simulink model "AMR_Testing_AutoMode_StateFlow"  (R2023b)
settings: Solver=FixedStepAuto  StartTime=0.0  StopTime=150  FixedStep=5e-3  RelTol=1e-3
model workspace (MAT data in the model file):
  RTK_health_condition = 30
  mdlWSDbList = ["C:\Users\matlab.cut\Desktop\AMR\canbus_files\tramontina_database_sick_modbus.dbc" "C:\Users\matlab.cut\Desktop\AMR\canbus_files\tramontina_database_xsens.dbc" "tramontina_database_curtis.dbc"]
  wheel_diameter = 360
  wheel_radius = 180
undefined symbols (not defined in the file or in its folder): Down, Pull
libraries: tramontina_database_xsenslib x4, speedgoatlib_IO60X_IO69X x2, tramontina_database_sick_modbuslib x1, speedgoatlib_IO691 x1, simulink_extras x1
settings Model: Creator=matlab.cut  LastModifiedBy=matlab.cut

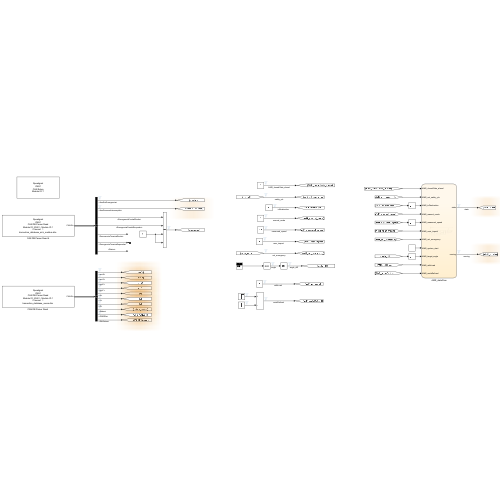
[thumbnail: Simulink's stored preview of the top-level diagram]
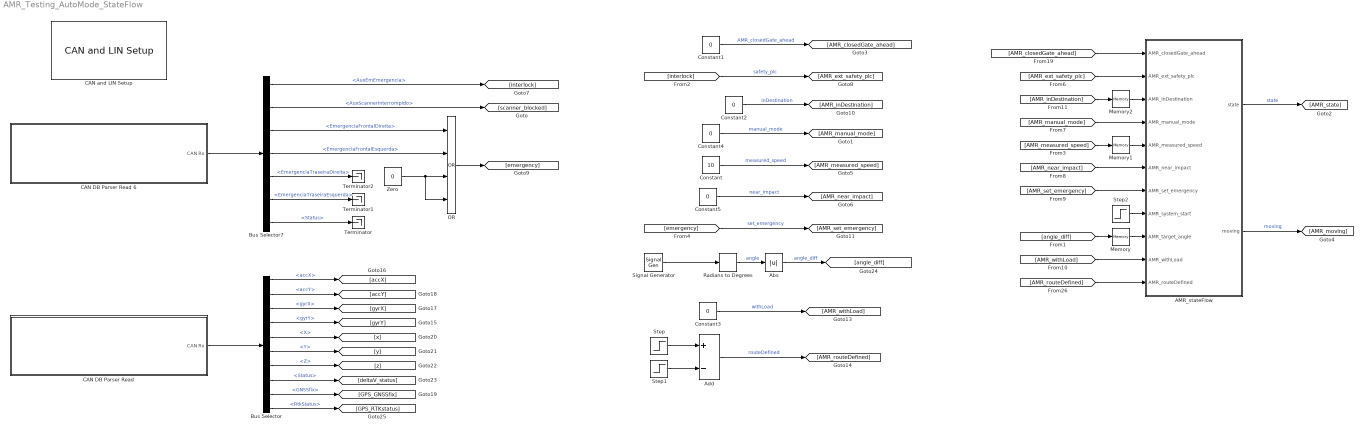
== system AMR_Testing_AutoMode_StateFlow ==
  AMR_stateFlow : Stateflow chart  TreatAsAtomicUnit=on
  Abs : Abs  SaturateOnIntegerOverflow=off
  Add : Sum  Inputs=+-
  Bus Selector : BusSelector  OutputSignals=ID52_Acceleration.accX,ID52_Acceleration.accY,ID50_RateOfTurn.gyrX,ID50_RateOfTurn.gyrY,ID49_DeltaV.X,ID49_DeltaV.Y,ID49_DeltaV.Z,ID49_DeltaV.MessageStatus.Status,ID17_StatusWord.GNSSfix,ID17_StatusWord.RtkStatus
  Bus Selector7 : BusSelector  OutputSignals=ID341_read_from_flexisoft.AuxEmEmergencia,ID341_read_from_flexisoft.AuxScannerInterrompido,ID341_read_from_flexisoft.EmergenciaFrontalDireita,ID341_read_from_flexisoft.EmergenciaFrontalEsquerda,ID341_read_from_flexisoft.EmergenciaTraseiraDireita,ID341_read_from_flexisoft.EmergenciaTraseiraEsquerda,ID341_read_from_flexisoft.MessageStatus.Status
  "CAN DB Parser Read " : Subsystem
      settings: OpenFcn=sg_can.OpenFcnRead;
      mask Help: eval('sg.utils.help.show(''io_main/refentry_ref_can_ofa_parsing_read'');')
      mask Display: disp('Speedgoat\nIO691\nCAN DB Parser Read\nModule ID: IO691 - Module ID 1\nChannel:  1\ntramontina_database_xsens.dbc ');
  CAN DB Parser Read 6 : Subsystem
      settings: OpenFcn=sg_can.OpenFcnRead;
      mask Help: eval('sg.utils.help.show(''io_main/refentry_ref_can_ofa_parsing_read'');')
      mask Display: disp('Speedgoat\nIO691\nCAN DB Parser Read\nModule ID: IO691 - Module ID 1\nChannel:  1\ntramontina_database_sick_modbus.dbc ');
  "CAN and LIN Setup " : speedgoatlib_IO691/CAN and LIN Setup   moduleInitValues="[691    1    1   -1   -1]"  id=1  moduleType=IO691  pciSlot=-1  canChn1=CAN (HS)  canChn2=Disabled  canChn3=Disabled  canChn4=Disabled  linChn1=Disabled  linChn2=Disabled  canInitStructArray=[]  canTermStructArray=[]  gpioChnx=Disabled  canChn1InitValues="[2   2   8   1  16   3  19   2   2   5   2   0]"  arbBdrChn1=500 kBaud  clockDividerChn1=Enable  arbManBdrChn1=[8,1,16,3]  fdBdrChn1=5.0 MBaud  fdManBdrChn1=[2,2,5,2]  termResistor1=off  canChn2InitValues="[1   0   2   8  31   8  19   2   2   5   2   0]"  arbBdrChn2=1.0 MBaud  clockDividerChn2=Enable  arbManBdrChn2=[2,8,31,8]  fdBdrChn2=5.0 MBaud  fdManBdrChn2=[2,2,5,2]  termResistor2=off  canChn3InitValues="[1   0   2   8  31   8  19   2   2   5   2   0]"  arbBdrChn3=1.0 MBaud  clockDividerChn3=Enable  arbManBdrChn3=[2,8,31,8]  fdBdrChn3=5.0 MBaud  fdManBdrChn3=[2,2,5,2]  termResistor3=off  canChn4InitValues="[1   0   2   8  31   8  19   2   2   5   2   0]"  arbBdrChn4=1.0 MBaud  clockDividerChn4=Enable  arbManBdrChn4=[2,8,31,8]  fdBdrChn4=5.0 MBaud  fdManBdrChn4=[2,2,5,2]  termResistor4=off  linChn1InitValues="[0  9600]"  linBtrChn1=9600  linChn2InitValues="[0  9600]"  linBtrChn2=9600  doInitTermStruct="[0  5  0  0  0]"  parDoChannels=[1 2]  parDoVoltage=5  parDoInitValues=0  parDoReset=1  parNumOfDoS=0  parDiChannels=[3 4]  parDiVoltage=5  parDiPull=Pull-Down
      settings: LibrarySourceBlock=speedgoatlib_IO602_IO691/CAN and LIN Setup
  Constant : Constant  Value=10
  Constant{1..5} (5 alike) : Constant  Value=0
  Memory : Memory
  Memory1 : Memory
  Memory2 : Memory
  OR : Logic  Operator=OR  Inputs=4  AllPortsSameDT=off  OutDataTypeStr=boolean
  Radians to Degrees : simulink_extras/Transformations/Radians to Degrees
  Signal Generator : SignalGenerator  Amplitude=0.1  Frequency=0.5
  Step : Step  Time=15  SampleTime=0
  Step1 : Step  Time=20  SampleTime=0
  Step2 : Step  Time=5  SampleTime=0
  Terminator : Terminator
  Terminator1 : Terminator
  Terminator2 : Terminator
  Zero : Constant  Value=0  OutDataTypeStr=Inherit: Inherit via back propagation
  wires:
  Memory/1 -> AMR_stateFlow/9(AMR_target_angle)
  Memory1/1 -> AMR_stateFlow/5(AMR_measured_speed)
  Step2/1 -> AMR_stateFlow/8(AMR_system_start)
  Memory2/1 -> AMR_stateFlow/3(AMR_inDestination)
  [AMR_routeDefined] -> AMR_stateFlow/11(AMR_routeDefined)
  [angle_diff] -> Memory/1
  [AMR_inDestination] -> Memory2/1
  [AMR_manual_mode] -> AMR_stateFlow/4(AMR_manual_mode)
  [AMR_near_impact] -> AMR_stateFlow/6(AMR_near_impact)
  [AMR_closedGate_ahead] -> AMR_stateFlow/1(AMR_closedGate_ahead)
  [AMR_measured_speed] -> Memory1/1
  AMR_stateFlow/2(moving) -> [AMR_moving]  "moving"
  [AMR_withLoad] -> AMR_stateFlow/10(AMR_withLoad)
  AMR_stateFlow/1(state) -> [AMR_state]  "state"
  [AMR_set_emergency] -> AMR_stateFlow/7(AMR_set_emergency)
  [AMR_ext_safety_plc] -> AMR_stateFlow/2(AMR_ext_safety_plc)
  Constant4/1 -> [AMR_manual_mode]  "manual_mode"
  Constant/1 -> [AMR_measured_speed]  "measured_speed"
  Constant5/1 -> [AMR_near_impact]  "near_impact"
  [interlock] -> [AMR_ext_safety_plc]  "safety_plc"
  Constant1/1 -> [AMR_closedGate_ahead]  "AMR_closedGate_ahead"
  Constant2/1 -> [AMR_inDestination]  "inDestination"
  [emergency] -> [AMR_set_emergency]  "set_emergency"
  Constant3/1 -> [AMR_withLoad]  "withLoad"
  Add/1 -> [AMR_routeDefined]  "routeDefined"
  Bus Selector7/5 -> Terminator2/1  "<EmergenciaTraseiraDireita>"
  Zero/1 -> OR/4, OR/3
  Bus Selector7/4 -> OR/2  "<EmergenciaFrontalEsquerda>"
  CAN DB Parser Read 6/1(CAN Rx) -> Bus Selector7/1
  Bus Selector7/7 -> Terminator/1  "<Status>"
  Bus Selector7/2 -> [scanner_blocked]  "<AuxScannerInterrompido>"
  Bus Selector7/6 -> Terminator1/1  "<EmergenciaTraseiraEsquerda>"
  Bus Selector7/3 -> OR/1  "<EmergenciaFrontalDireita>"
  Bus Selector7/1 -> [interlock]  "<AuxEmEmergencia>"
  OR/1 -> [emergency]
  Step1/1 -> Add/2
  Step/1 -> Add/1
  Bus Selector/10 -> [GPS_RTKstatus]  "<RtkStatus>"
  "CAN DB Parser Read "/1(CAN Rx) -> Bus Selector/1
  Bus Selector/3 -> [gyrX]  "<gyrX>"
  Bus Selector/2 -> [accY]  "<accY>"
  Bus Selector/4 -> [gyrY]  "<gyrY>"
  Bus Selector/1 -> [accX]  "<accX>"
  Bus Selector/9 -> [GPS_GNSSfix]  "<GNSSfix>"
  Bus Selector/5 -> [x]  "<X>"
  Bus Selector/6 -> [y]  "<Y>"
  Bus Selector/7 -> [z]  "<Z>"
  Bus Selector/8 -> [deltaV_status]  "<Status>"
  Abs/1 -> [angle_diff]  "angle_diff"
  Signal Generator/1 -> Radians to Degrees/1
  Radians to Degrees/1 -> Abs/1  "angle"

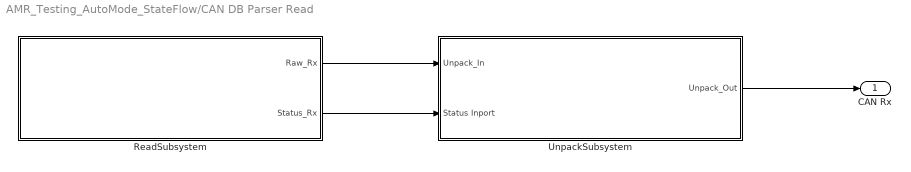
== system AMR_Testing_AutoMode_StateFlow/CAN DB Parser Read  ==
  ReadSubsystem : Subsystem
  UnpackSubsystem : Subsystem
  CAN Rx : Outport
  wires:
  ReadSubsystem/1(Raw_Rx) -> UnpackSubsystem/1(Unpack_In)
  ReadSubsystem/2(Status_Rx) -> UnpackSubsystem/2(Status Inport)
  UnpackSubsystem/1(Unpack_Out) -> CAN Rx/1

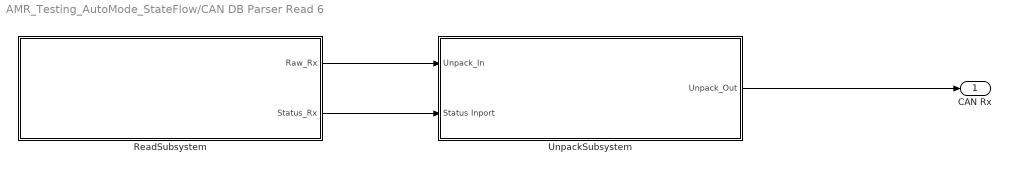
== system AMR_Testing_AutoMode_StateFlow/CAN DB Parser Read 6 ==
  ReadSubsystem : Subsystem
  UnpackSubsystem : Subsystem
  CAN Rx : Outport
  wires:
  ReadSubsystem/1(Raw_Rx) -> UnpackSubsystem/1(Unpack_In)
  ReadSubsystem/2(Status_Rx) -> UnpackSubsystem/2(Status Inport)
  UnpackSubsystem/1(Unpack_Out) -> CAN Rx/1

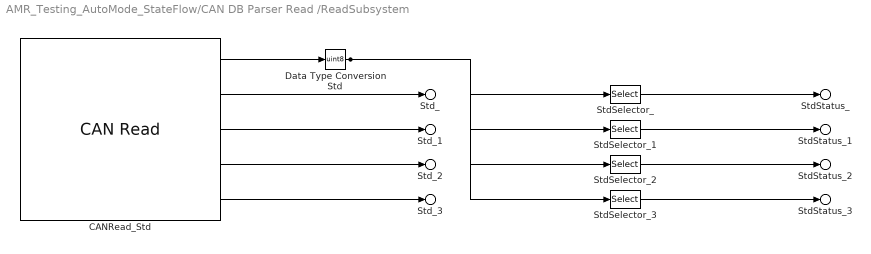
== system AMR_Testing_AutoMode_StateFlow/CAN DB Parser Read /ReadSubsystem ==
  CANRead_Std : speedgoatlib_IO60X_IO69X/CAN/CAN Read   moduleType=IO691  id=1  channel=1  canType=CAN (HS)  messageType=CAN (HS)  useBusOut=on  HasMulRead=Specify by IDs  MsgIDlist="[17  49  50  52]"  isEFF=off  LabelInHex=off  enableInput=off  initValues=[691 1 0.01 0 1 1 0 1 2 0 4 17 49 50 52]  ts=10e-3
  Data Type ConversionStd : DataTypeConversion  OutDataTypeStr=uint8  SaturateOnIntegerOverflow=off  RndMeth=Floor
  StdSelector_ : Selector  IndexOptions=Index vector (dialog)  Indices=1  OutputSizes=1
  StdSelector_1 : Selector  IndexOptions=Index vector (dialog)  Indices=2  OutputSizes=1
  StdSelector_2 : Selector  IndexOptions=Index vector (dialog)  Indices=3  OutputSizes=1
  StdSelector_3 : Selector  IndexOptions=Index vector (dialog)  Indices=4  OutputSizes=1
  Std_ : Outport  PortName=Raw_Rx  Element=Std.ID17
  Std_1 : Outport  PortName=Raw_Rx  Element=Std.ID49
  Std_2 : Outport  PortName=Raw_Rx  Element=Std.ID50
  Std_3 : Outport  PortName=Raw_Rx  Element=Std.ID52
  StdStatus_ : Outport  Port=2  PortName=Status_Rx  Element=Std.ID17
  StdStatus_1 : Outport  Port=2  PortName=Status_Rx  Element=Std.ID49
  StdStatus_2 : Outport  Port=2  PortName=Status_Rx  Element=Std.ID50
  StdStatus_3 : Outport  Port=2  PortName=Status_Rx  Element=Std.ID52
  wires:
  CANRead_Std/1 -> Data Type ConversionStd/1
  CANRead_Std/2 -> Std_/1
  CANRead_Std/3 -> Std_1/1
  CANRead_Std/4 -> Std_2/1
  CANRead_Std/5 -> Std_3/1
  Data Type ConversionStd/1 -> StdSelector_/1, StdSelector_1/1, StdSelector_2/1, StdSelector_3/1
  StdSelector_/1 -> StdStatus_/1
  StdSelector_1/1 -> StdStatus_1/1
  StdSelector_2/1 -> StdStatus_2/1
  StdSelector_3/1 -> StdStatus_3/1

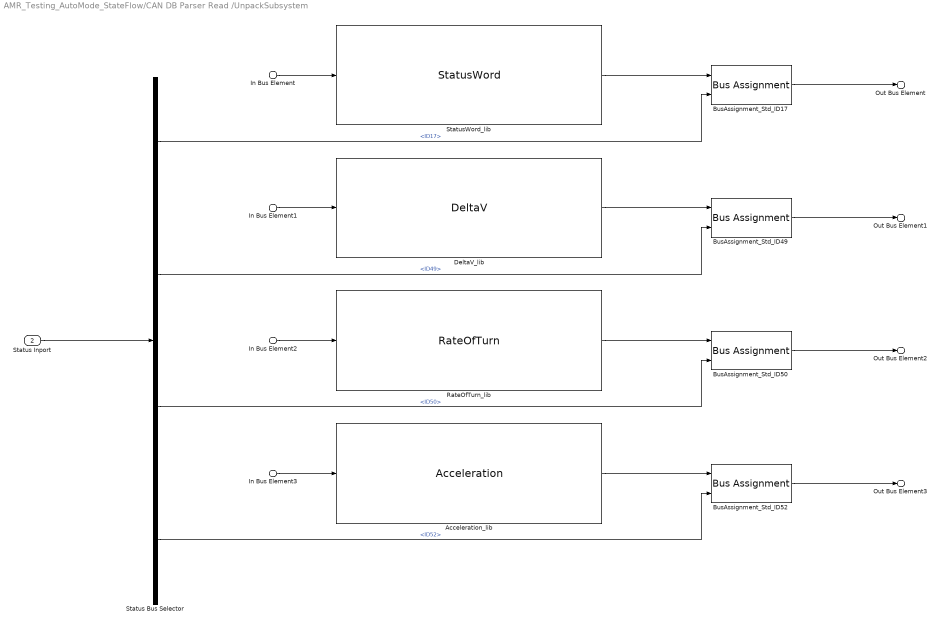
== system AMR_Testing_AutoMode_StateFlow/CAN DB Parser Read /UnpackSubsystem ==
  In Bus Element : Inport  PortName=Unpack_In  Element=Std.ID17
  In Bus Element1 : Inport  PortName=Unpack_In  Element=Std.ID49
  In Bus Element2 : Inport  PortName=Unpack_In  Element=Std.ID50
  In Bus Element3 : Inport  PortName=Unpack_In  Element=Std.ID52
  Status Inport : Inport  Port=2
  Acceleration_lib : tramontina_database_xsenslib/CAN unpack/Acceleration  SystemSampleTime=-1  VariantActivationTime=update diagram  AllowFlexibleInterface=on  Latency=0  AutoFrameSizeCalculation=off
  BusAssignment_Std_ID{17,49..50,52} (4 alike) : BusAssignment  AssignedSignals=MessageStatus.Status
  DeltaV_lib : tramontina_database_xsenslib/CAN unpack/DeltaV  SystemSampleTime=-1  VariantActivationTime=update diagram  AllowFlexibleInterface=on  Latency=0  AutoFrameSizeCalculation=off
  RateOfTurn_lib : tramontina_database_xsenslib/CAN unpack/RateOfTurn  SystemSampleTime=-1  VariantActivationTime=update diagram  AllowFlexibleInterface=on  Latency=0  AutoFrameSizeCalculation=off
  Status Bus Selector : BusSelector  OutputSignals=Std.ID17,Std.ID49,Std.ID50,Std.ID52
  StatusWord_lib : tramontina_database_xsenslib/CAN unpack/StatusWord  SystemSampleTime=-1  VariantActivationTime=update diagram  AllowFlexibleInterface=on  Latency=0  AutoFrameSizeCalculation=off
  Out Bus Element : Outport  PortName=Unpack_Out  Element=ID17_StatusWord
  Out Bus Element1 : Outport  PortName=Unpack_Out  Element=ID49_DeltaV
  Out Bus Element2 : Outport  PortName=Unpack_Out  Element=ID50_RateOfTurn
  Out Bus Element3 : Outport  PortName=Unpack_Out  Element=ID52_Acceleration
  wires:
  In Bus Element/1 -> StatusWord_lib/1
  StatusWord_lib/1 -> BusAssignment_Std_ID17/1
  BusAssignment_Std_ID17/1 -> Out Bus Element/1
  In Bus Element1/1 -> DeltaV_lib/1
  DeltaV_lib/1 -> BusAssignment_Std_ID49/1
  BusAssignment_Std_ID49/1 -> Out Bus Element1/1
  In Bus Element2/1 -> RateOfTurn_lib/1
  RateOfTurn_lib/1 -> BusAssignment_Std_ID50/1
  BusAssignment_Std_ID50/1 -> Out Bus Element2/1
  In Bus Element3/1 -> Acceleration_lib/1
  Acceleration_lib/1 -> BusAssignment_Std_ID52/1
  BusAssignment_Std_ID52/1 -> Out Bus Element3/1
  Status Inport/1 -> Status Bus Selector/1
  Status Bus Selector/1 -> BusAssignment_Std_ID17/2  "<ID17>"
  Status Bus Selector/2 -> BusAssignment_Std_ID49/2  "<ID49>"
  Status Bus Selector/3 -> BusAssignment_Std_ID50/2  "<ID50>"
  Status Bus Selector/4 -> BusAssignment_Std_ID52/2  "<ID52>"

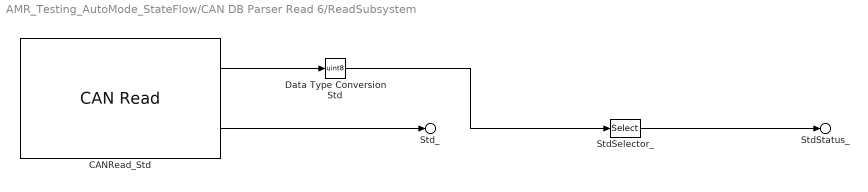
== system AMR_Testing_AutoMode_StateFlow/CAN DB Parser Read 6/ReadSubsystem ==
  CANRead_Std : speedgoatlib_IO60X_IO69X/CAN/CAN Read   moduleType=IO691  id=1  channel=1  canType=CAN (HS)  messageType=CAN (HS)  useBusOut=on  HasMulRead=Specify by IDs  MsgIDlist=[341]  isEFF=off  LabelInHex=off  enableInput=off  initValues=[691 1 0.1 0 1 1 0 1 2 0 1 341]  ts=100e-3
  Data Type ConversionStd : DataTypeConversion  OutDataTypeStr=uint8  SaturateOnIntegerOverflow=off  RndMeth=Floor
  StdSelector_ : Selector  IndexOptions=Index vector (dialog)  Indices=1  OutputSizes=1
  Std_ : Outport  PortName=Raw_Rx  Element=Std.ID341
  StdStatus_ : Outport  Port=2  PortName=Status_Rx  Element=Std.ID341
  wires:
  CANRead_Std/1 -> Data Type ConversionStd/1
  CANRead_Std/2 -> Std_/1
  Data Type ConversionStd/1 -> StdSelector_/1
  StdSelector_/1 -> StdStatus_/1

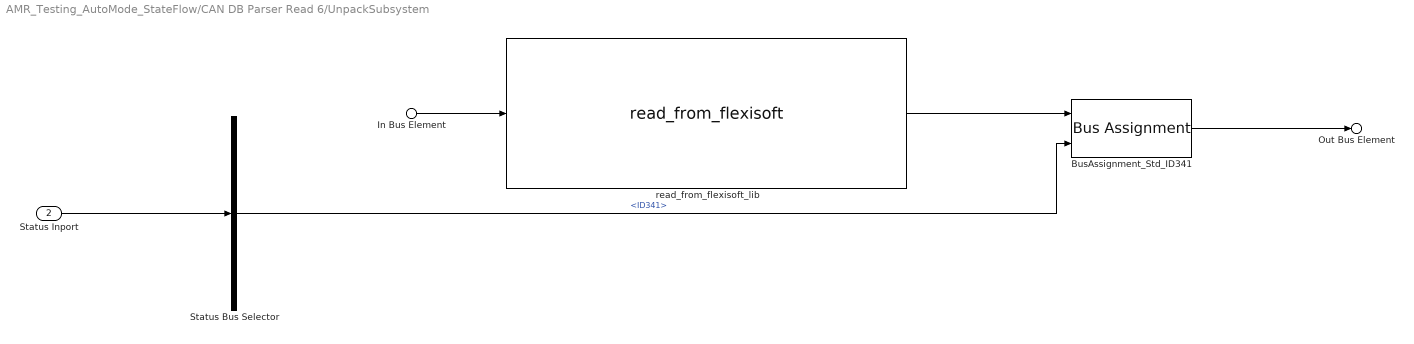
== system AMR_Testing_AutoMode_StateFlow/CAN DB Parser Read 6/UnpackSubsystem ==
  In Bus Element : Inport  PortName=Unpack_In  Element=Std.ID341
  Status Inport : Inport  Port=2
  BusAssignment_Std_ID341 : BusAssignment  AssignedSignals=MessageStatus.Status
  Status Bus Selector : BusSelector  OutputSignals=Std.ID341
  read_from_flexisoft_lib : tramontina_database_sick_modbuslib/CAN unpack/read_from_flexisoft  SystemSampleTime=-1  VariantActivationTime=update diagram  AllowFlexibleInterface=on  Latency=0  AutoFrameSizeCalculation=off
  Out Bus Element : Outport  PortName=Unpack_Out  Element=ID341_read_from_flexisoft
  wires:
  In Bus Element/1 -> read_from_flexisoft_lib/1
  read_from_flexisoft_lib/1 -> BusAssignment_Std_ID341/1
  BusAssignment_Std_ID341/1 -> Out Bus Element/1
  Status Inport/1 -> Status Bus Selector/1
  Status Bus Selector/1 -> BusAssignment_Std_ID341/2  "<ID341>"

== stateflow chart AMR_Testing_AutoMode_StateFlow/AMR_stateFlow ==
  note: Constantes:
      | WAITING = 0
      | SUCCESS=1
      | FAIL=-1
      | FALSE=0
      | TRUE=1
      |
      | Flags:
      | AMR_speed_measued = double() => Captura a velocidade do AMR
      | AMR_target_angle = double() => Captura o ângulo entre o AMR e o próximo waypoing
      | AMR_near_impact = TRUE => Sensor acusa impacto iminente
      | AMR_near_impact = FALSE => Sensor de impacto diz que está livre
      | AMR_ext_safety_plc = TRUE => Estado de emergência foi resolvido
      | AMR_ext_safety_plc = FALSE => Estado de emergência não foi resolvido
      | AMR_closedGate_ahead = TRUE => Existe um portão fechado a frente
      | AMR_closedGate_ahead = FALSE => Caminho livre
      | AMR_withLoad = TRUE => AMR está com carga (segue para estado de unloading)
      | AMR_withLoad = FALSE => AMR está sem carga (segue para o estado de loading)
      | AMR_inDestination = TRUE => AMR chegou ao destino de carga ou descarga
      | AMR_inDestination = FAIL => AMR chegou ao destino de carga ou descarga
      | AMR_system_startup = WAITING => AMR não foi inicializado (aguardando)
      | AMR_system_startup = SUCCESS => AMR inicializado com sucesso
      | AMR_system_startup = FAIL => AMR inicializado com falha
      | AMR_system_emergency = TRUE => AMR vai para modo de emergência
      | AMR_system_emergency = FALSE => AMR continua sua operação normal
      | AMR_manual_mode = TRUE => AMR vai para modo manual
      | AMR_manual_mode = FALSE => AMR continua sua operação normal
      | AMR_routeDefined = TRUE => AMR com rota definida
      | AMR_routeDefined = FALSE => AMR sem rota definida
  state S0_startup
    entry:
    state = 0;
    moving = 0;
    settings: description=This state models the modes of a window sensor and implements logic to respond when that sensor is producing a signal.
  state E1_failed
    entry:
    state = -1;
    moving = 0;
    settings: description=This state models the modes of a window sensor and implements logic to respond when that sensor is producing a signal.
  state autonomousOperation
    settings: description=This state models the modes of a window sensor and implements logic to respond when that sensor is producing a signal.
    state S2_engaged
      entry:
      state = 2;
      settings: description=This state models the modes of a window sensor and implements logic to respond when that sensor is producing a signal.
      state S2A_Rotation
        entry:
        moving = 1;
      state S2B_Moving
        entry:
        moving = 2;
      state S2C_Parking
        entry:
        moving = 3;
      state S2D_Stopped
        entry:
        moving = 0;
      state S2E_Gate
        entry:
        moving = 0;
      (default) -> S2A_Rotation
      S2B_Moving -> (junction 285) [order 1] : [AMR_near_impact == TRUE]
      (junction 285) -> (junction 290)
      S2A_Rotation -> S2B_Moving : [AMR_target_angle <= 15]
      S2B_Moving -> S2C_Parking [order 2] : [AMR_target_angle > 15 | AMR_closedGate_ahead==TRUE | AMR_inDestination == TRUE]
      (junction 300) -> S2A_Rotation
      S2C_Parking -> (junction 290) [order 1] : [AMR_near_impact == TRUE]
      (junction 290) -> (junction 286)
      (junction 299) -> (junction 300)
      S2E_Gate -> (junction 300) [order 2] : [AMR_closedGate_ahead==TRUE]
      (junction 295) -> (junction 299) [order 3]
      S2C_Parking -> S2D_Stopped [order 2] : [AMR_measured_speed < 0.05]
      S2E_Gate -> S2E_Gate [order 1] : after(60, sec)
      (junction 295) -> S2E_Gate [order 2] : [AMR_closedGate_ahead==TRUE]
      S2D_Stopped -> (junction 295) : [AMR_near_impact == FALSE && AMR_measured_speed < 0.05]
      (junction 286) -> S2D_Stopped
    state S1_standby
      entry:
      state = 1;
      settings: description=This state models the modes of a window sensor and implements logic to respond when that sensor is producing a signal.
    state S4_unloading
      entry:
      state = 4;
      settings: description=This state models the modes of a window sensor and implements logic to respond when that sensor is producing a signal.
    state S3_loading
      entry:
      state = 3;
      settings: description=This state models the modes of a window sensor and implements logic to respond when that sensor is producing a signal.
    (default) -> S1_standby
    S1_standby -> S2_engaged : [AMR_routeDefined == TRUE]
    S4_unloading -> S1_standby
    (junction 269) -> S2_engaged
    S3_loading -> (junction 269)
    (junction 295) -> (junction 253) [order 1] : [AMR_inDestination==TRUE]
    (junction 275) -> S4_unloading
    (junction 254) -> S3_loading [order 1] : [AMR_withLoad == FALSE]
    (junction 254) -> (junction 275) [order 2] : [AMR_withLoad == TRUE]
    (junction 253) -> (junction 254)
  state E2_emergency
    entry:
    state = -2;
    moving = 0;
    settings: description=This state models the modes of a window sensor and implements logic to respond when that sensor is producing a signal.
  state E3_manualMode
    entry:
    state = -3;
    moving = 0;
    settings: description=This state models the modes of a window sensor and implements logic to respond when that sensor is producing a signal.
  (default) -> (junction 244)
  (junction 242) -> (junction 244)
  (junction 244) -> S0_startup
  (junction 312) -> (junction 242)
  S0_startup -> (junction 257) : [AMR_system_start ~= WAITING]
  (junction 257) -> (junction 251) [order 1] : [AMR_system_start == FAIL]
  (junction 257) -> autonomousOperation [order 2] : [AMR_system_start == SUCCESS]
  (junction 251) -> E1_failed
  autonomousOperation -> E1_failed [order 3] : [AMR_system_start == FAIL]
  E1_failed -> (junction 312)
  (junction 243) -> (junction 312)
  E2_emergency -> (junction 243) [order 1] : [AMR_ext_safety_plc == TRUE]
  autonomousOperation -> E2_emergency [order 1] : [AMR_set_emergency == TRUE]
  E2_emergency -> E2_emergency [order 2] : after(10, sec)
  autonomousOperation -> E3_manualMode [order 2] : [AMR_manual_mode == TRUE]
  E3_manualMode -> autonomousOperation : [AMR_manual_mode == FALSE]
  data: state output =0; moving output; FAIL constant double =-1; SUCCESS constant double =1; WAITING constant double =0; AMR_closedGate_ahead input; AMR_ext_safety_plc input; AMR_inDestination input; AMR_manual_mode input; AMR_measured_speed input; AMR_near_impact input; AMR_set_emergency input; AMR_system_start input; AMR_target_angle input; AMR_withLoad input; FALSE constant double =0; TRUE constant double =1; AMR_routeDefined input
